simulink model "test4"  (R2016a)
settings: Solver=VariableStepAuto  StartTime=0.0  StopTime=10.0  RelTol=1e-3
libraries: powerlib x13, powerlib_meascontrol x1, simulink x1
settings Model: Creator=Dang Khoa  LastModifiedBy=Dang Khoa

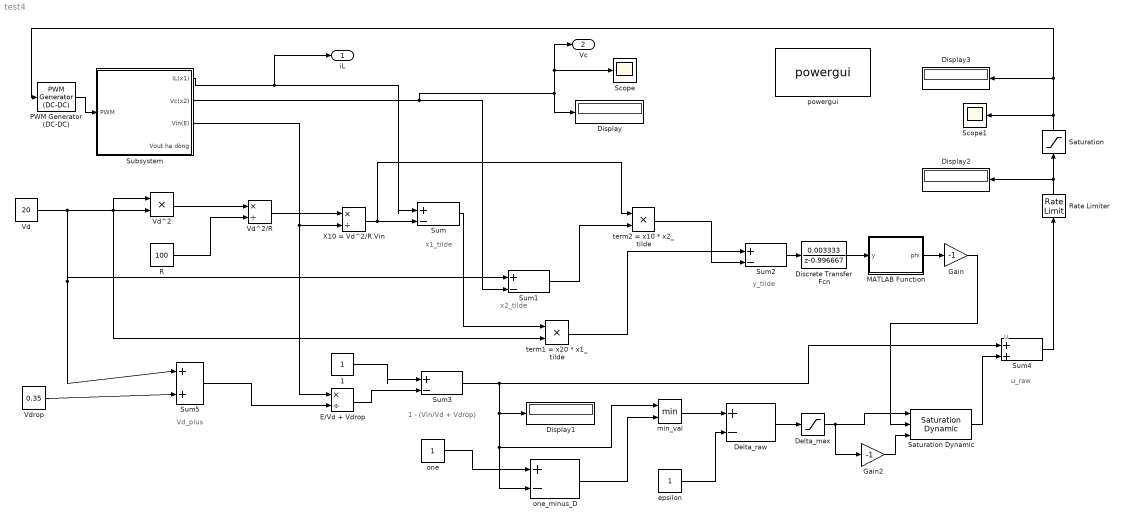
== system test4 ==
  note: Vd_plus
  note: u_raw
  note: u
  note: 1 - (Vin/Vd + Vdrop)
  note: x1_tilde
  note: x2_tilde
  note: y_tilde
  "1 " : Constant
  Delta_max : Saturate  UpperLimit=inf  LowerLimit=0
  Delta_raw : Sum  Inputs=+-
  Discrete Transfer Fcn : DiscreteTransferFcn  Numerator=[0.003333]  Denominator=[1 -0.996667]  SampleTime=5e-6
  Display{,1..3} (4 alike) : Display
  E/Vd + Vdrop : Product  Inputs=*/
  Gain : Gain  Gain=-1
  Gain2 : Gain  Gain=-1
  MATLAB Function : MATLAB Function  TreatAsAtomicUnit=on
  PWM Generator (DC-DC) : powerlib_meascontrol/Pulse & Signal Generators/PWM Generator (DC-DC)  Fsw=20000  Ts=5e-6
  R : Constant  Value=100
  Rate Limiter : RateLimiter  RisingSlewLimit=0.5  FallingSlewLimit=-0.5  SampleTimeMode=inherited
  Saturation : Saturate  UpperLimit=1  LowerLimit=0
  Saturation Dynamic : simulink/Discontinuities/Saturation Dynamic  OutMin=[]  OutMax=[]  OutDataTypeStr=Inherit: Same as second input  OutDataType=fixdt(1, 16)  OutScaling=2^-10  DoSatur=off
  Scope : Scope
  Scope1 : Scope
  Subsystem : Subsystem
  Sum{,1..3} (4 alike) : Sum  Inputs=|+-
  Sum4 : Sum  Inputs=|++
  Sum5 : Sum  Inputs=|++
  Vd : Constant  Value=20
  Vd^2 : Product
  Vd^2/R : Product  Inputs=*/
  Vdrop : Constant  Value=0.35
  X10 = Vd^2/R.Vin : Product  Inputs=*/
  epsilon : Constant
  min_val : MinMax  Inputs=2
  one : Constant
  one_minus_D : Sum  Inputs=+-
  powergui : powerlib/powergui  Priority=1  SimulationMode=Discrete  SolverType=Tustin/Backward Euler (TBE)  SampleTime=5e-6  frequency=60  SPID=off  DisableSnubberDevices=off  DisableRonSwitches=off  DisableVfSwitches=off  SwTol=0  DisplayEquations=off  Interpol=off  ExternalGateDelay=off  methode=off  Ts=10  FunctionMessages=off  echomessages=off  HookPort=off  EnableUseOfTLC=off  x0status=blocks  frequencyindice=0  Pbase=100e6  ErrMax=1e-4  Iterations=50  UnitsV=kV  UnitsW=MW  buscounter=0  RestoreLinks=warning  ResistiveCurrentMeasurement=off  Frange=[0:2:500]  Ylog=off  Xlog=on  ShowGrid=off  save=off  variable=ZData  structure=0  ZoomFFT=off  StartTime=0.0  cycles=1  DisplayStyle=1  fundamental=60  FreqAxis=off  MaxFrequency=1000  frequencyindicesteady=1  RmsSteady=1  display=off
  term1 = x20 * x1_tilde : Product
  term2 = x10 * x2_tilde : Product
  iL : Outport
  Vc : Outport  Port=2
  wires:
  PWM Generator (DC-DC)/1 -> Subsystem/1(PWM)
  Subsystem/1(iL(x1)) -> iL/1, Sum/1
  Vd/1 -> Sum1/1, Sum5/1, term1 = x20 * x1_tilde/2, Vd^2/1, Vd^2/2
  Vd^2/1 -> Vd^2/R/1
  R/1 -> Vd^2/R/2
  Vd^2/R/1 -> X10 = Vd^2/R.Vin/1
  Subsystem/3(Vin(E)) -> E/Vd + Vdrop/1, X10 = Vd^2/R.Vin/2
  X10 = Vd^2/R.Vin/1 -> term2 = x10 * x2_tilde/1, Sum/2
  Subsystem/2(Vc(x2)) -> Vc/1, Scope/1, Display/1, Sum1/2
  Sum/1 -> term1 = x20 * x1_tilde/1
  Sum1/1 -> term2 = x10 * x2_tilde/2
  term1 = x20 * x1_tilde/1 -> Sum2/1
  term2 = x10 * x2_tilde/1 -> Sum2/2
  MATLAB Function/1(phi) -> Gain/1
  "1 "/1 -> Sum3/1
  E/Vd + Vdrop/1 -> Sum3/2
  Sum3/1 -> Sum4/1, min_val/1, one_minus_D/2, Display1/1
  one/1 -> one_minus_D/1
  one_minus_D/1 -> min_val/2
  min_val/1 -> Delta_raw/1
  epsilon/1 -> Delta_raw/2
  Delta_raw/1 -> Delta_max/1
  Delta_max/1 -> Gain2/1, Saturation Dynamic/1
  Gain2/1 -> Saturation Dynamic/3
  Saturation Dynamic/1 -> Sum4/2
  Gain/1 -> Saturation Dynamic/2
  Sum2/1 -> Discrete Transfer Fcn/1
  Discrete Transfer Fcn/1 -> MATLAB Function/1(y)
  Vdrop/1 -> Sum5/2
  Sum5/1 -> E/Vd + Vdrop/2
  Sum4/1 -> Rate Limiter/1
  Rate Limiter/1 -> Saturation/1, Display2/1
  Saturation/1 -> Display3/1, PWM Generator (DC-DC)/1, Scope1/1

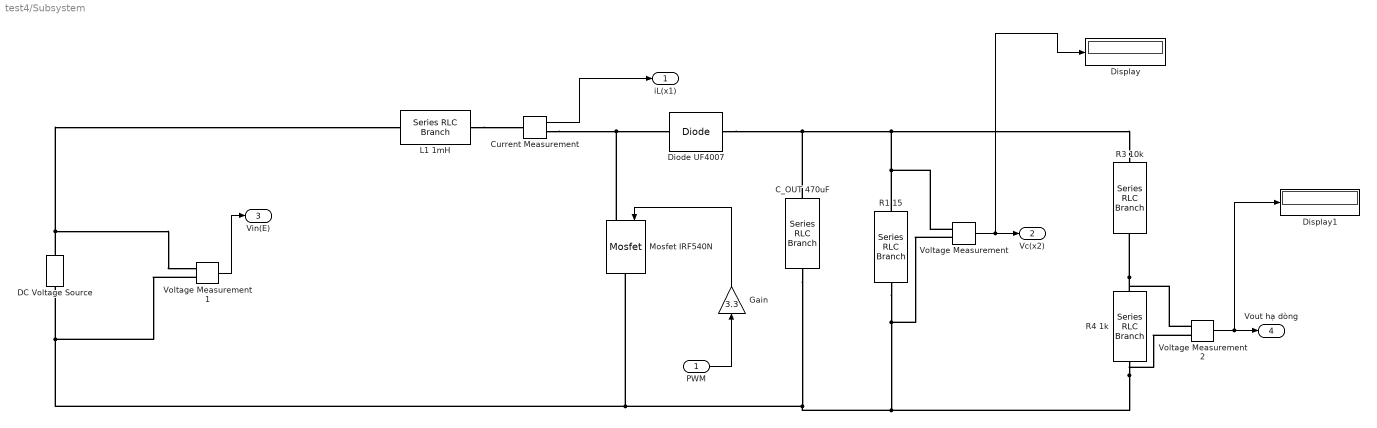
== system test4/Subsystem ==
  PWM : Inport
  C_OUT 470uF : powerlib/Elements/Series RLC Branch  LConnTagsString=__new0  RConnTagsString=__new0  BranchType=C  Resistance=1  Inductance=1e-3  SetiL0=off  InitialCurrent=0  Capacitance=470e-6  Setx0=off  InitialVoltage=0  Measurements=None
  Current Measurement : powerlib/Measurements/Current Measurement  PhasorSimulation=off  OutputType=Complex  PSBequivalent=0
  DC Voltage Source : powerlib/Electrical Sources/DC Voltage Source  Amplitude=15  Measurements=None
  Diode UF4007 : powerlib/Power Electronics/Diode  Ron=0.05  Lon=0  Vf=1  IC=0  UseSnubber=off  Rs=500  Cs=250e-12  Measurements=off
  Display : Display
  Display1 : Display
  Gain : Gain  Gain=3.3
  L1 1mH : powerlib/Elements/Series RLC Branch  LConnTagsString=__new0  RConnTagsString=__new0  BranchType=L  Resistance=1  Inductance=0.001  SetiL0=off  InitialCurrent=0  Capacitance=1e-6  Setx0=off  InitialVoltage=0  Measurements=None
  Mosfet IRF540N : powerlib/Power Electronics/Mosfet  Ron=0.02  Lon=0  Rd=0.03  Vfd=1  IC=0  Rs=inf  Cs=inf  Measurements=off
  R1 15 : powerlib/Elements/Series RLC Branch  LConnTagsString=__new0  RConnTagsString=__new0  BranchType=R  Resistance=15  Inductance=1e-3  SetiL0=off  InitialCurrent=0  Capacitance=1e-6  Setx0=off  InitialVoltage=0  Measurements=None
  R3 10k : powerlib/Elements/Series RLC Branch  LConnTagsString=__new0  RConnTagsString=__new0  BranchType=R  Resistance=100000  Inductance=1e-3  SetiL0=off  InitialCurrent=0  Capacitance=1e-6  Setx0=off  InitialVoltage=0  Measurements=None
  R4 1k : powerlib/Elements/Series RLC Branch  LConnTagsString=__new0  RConnTagsString=__new0  BranchType=R  Resistance=10000  Inductance=1e-3  SetiL0=off  InitialCurrent=0  Capacitance=1e-6  Setx0=off  InitialVoltage=0  Measurements=None
  Voltage Measurement : powerlib/Measurements/Voltage Measurement  PhasorSimulation=off  OutputType=Complex  PSBequivalent=0
  Voltage Measurement1 : powerlib/Measurements/Voltage Measurement  PhasorSimulation=off  OutputType=Complex  PSBequivalent=0
  Voltage Measurement2 : powerlib/Measurements/Voltage Measurement  PhasorSimulation=off  OutputType=Complex  PSBequivalent=0
  iL(x1) : Outport
  Vc(x2) : Outport  Port=2
  Vin(E) : Outport  Port=3
  Vout hạ dòng : Outport  Port=4
  wires:
  Voltage Measurement/1 -> Display/1, Vc(x2)/1
  Voltage Measurement1/1 -> Vin(E)/1
  Current Measurement/1 -> iL(x1)/1
  PWM/1 -> Gain/1
  Gain/1 -> Mosfet IRF540N/1
  Voltage Measurement2/1 -> Display1/1, Vout hạ dòng/1
  connections:
  R4 1k/LConn1 -- R3 10k/RConn1 -- Voltage Measurement2/LConn1
  Mosfet IRF540N/LConn1 -- Current Measurement/RConn1 -- Diode UF4007/LConn1
  R1 15/LConn1 -- Voltage Measurement/LConn1 -- R3 10k/LConn1 -- C_OUT 470uF/LConn1 -- Diode UF4007/RConn1
  L1 1mH/RConn1 -- Current Measurement/LConn1
  DC Voltage Source/RConn1 -- L1 1mH/LConn1 -- Voltage Measurement1/LConn1
  C_OUT 470uF/RConn1 -- Voltage Measurement2/LConn2 -- R4 1k/RConn1 -- R1 15/RConn1 -- Voltage Measurement/LConn2 -- Voltage Measurement1/LConn2 -- DC Voltage Source/LConn1 -- Mosfet IRF540N/RConn1

== matlab function test4/MATLAB Function ==
  data: y input; phi output
function phi = PBCphi(y)
a1 = 1; 
a2 = 0.5; 
a3 = 0.02;   % đúng PL2, bạn giữ/tune được
phi = a1*y + a2*y^3 + a3*y^5;
end
